simulink model "ControlSystem"  (R2022a)
settings: Solver=FixedStepAuto  StartTime=0.0  StopTime=35  FixedStep=0.01  RelTol=0.01
InitFcn:
  | C=4200;
undefined symbols (not defined in the file): xpoints, ypoints
libraries: simulink_extras x2
settings Model: NumberOfSteps=1100  Creator=tumu  LastModifiedBy=tumu
settings SolverCC: AlgebraicLoopSolver=TrustRegion
settings DebuggingCC: UnconnectedInputMsg=warning  UnconnectedOutputMsg=warning  UnconnectedLineMsg=warning  SFMachineParentedDataDiag=warning  UnderSpecifiedDimensionMsg=warning
settings ModelReferenceCC: ModelReferenceNumInstancesAllowed=Single

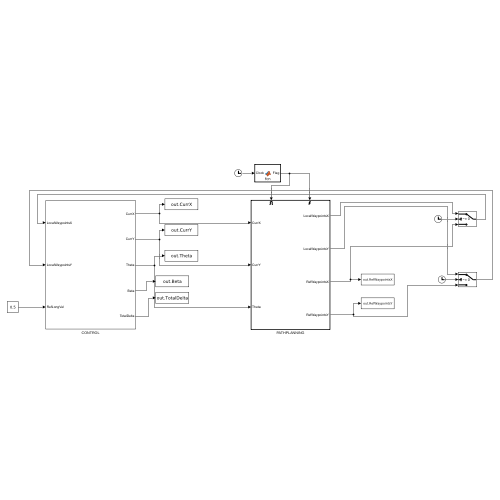
[thumbnail: Simulink's stored preview of the top-level diagram]
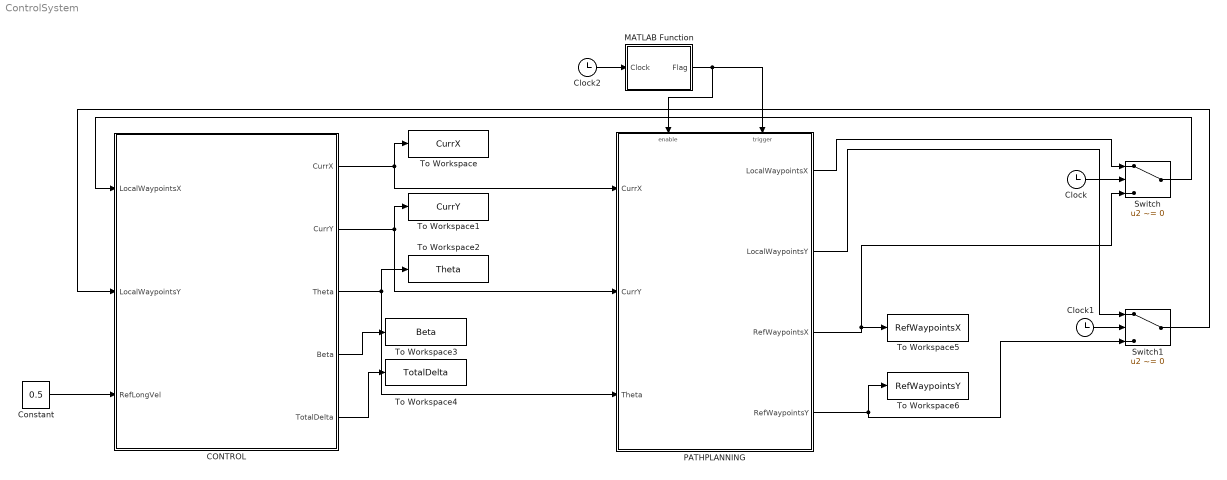
== system ControlSystem ==
  CONTROL : Subsystem
  Clock : Clock
  Clock1 : Clock
  Clock2 : Clock
  Constant : Constant  Value=0.5
  MATLAB Function : MATLAB Function  TreatAsAtomicUnit=on
  PATHPLANNING : Subsystem
  Switch : Switch  Criteria=u2 ~= 0  SaturateOnIntegerOverflow=off  InputSameDT=off
  Switch1 : Switch  Criteria=u2 ~= 0  SaturateOnIntegerOverflow=off  InputSameDT=off
  To Workspace : ToWorkspace  VariableName=CurrX  SaveFormat=Structure With Time  SampleTime=-1
  To Workspace1 : ToWorkspace  VariableName=CurrY  SaveFormat=Structure With Time  SampleTime=-1
  To Workspace2 : ToWorkspace  VariableName=Theta  SaveFormat=Structure With Time  SampleTime=-1
  To Workspace3 : ToWorkspace  VariableName=Beta  SaveFormat=Structure With Time  SampleTime=-1
  To Workspace4 : ToWorkspace  VariableName=TotalDelta  SaveFormat=Structure With Time  SampleTime=-1
  To Workspace5 : ToWorkspace  VariableName=RefWaypointsX  SampleTime=-1
      settings: Save2DSignal=2-D array (concatenate along first dimension)
  To Workspace6 : ToWorkspace  VariableName=RefWaypointsY  SampleTime=-1
      settings: Save2DSignal=2-D array (concatenate along first dimension)
  wires:
  CONTROL/2(CurrY) -> To Workspace1/1, PATHPLANNING/2(CurrY)
  CONTROL/3(Theta) -> To Workspace2/1, PATHPLANNING/3(Theta)
  CONTROL/4(Beta) -> To Workspace3/1
  CONTROL/5(TotalDelta) -> To Workspace4/1
  CONTROL/1(CurrX) -> To Workspace/1, PATHPLANNING/1(CurrX)
  PATHPLANNING/1(LocalWaypointsX) -> Switch/1
  Clock2/1 -> MATLAB Function/1(Clock)
  MATLAB Function/1(Flag) -> PATHPLANNING/Trigger, PATHPLANNING/Enable
  PATHPLANNING/3(RefWaypointsX) -> To Workspace5/1, Switch/3
  PATHPLANNING/4(RefWaypointsY) -> Switch1/3, To Workspace6/1
  Clock/1 -> Switch/2
  Switch/1 -> CONTROL/1(LocalWaypointsX)
  Clock1/1 -> Switch1/2
  Switch1/1 -> CONTROL/2(LocalWaypointsY)
  PATHPLANNING/2(LocalWaypointsY) -> Switch1/1
  Constant/1 -> CONTROL/3(RefLongVel)

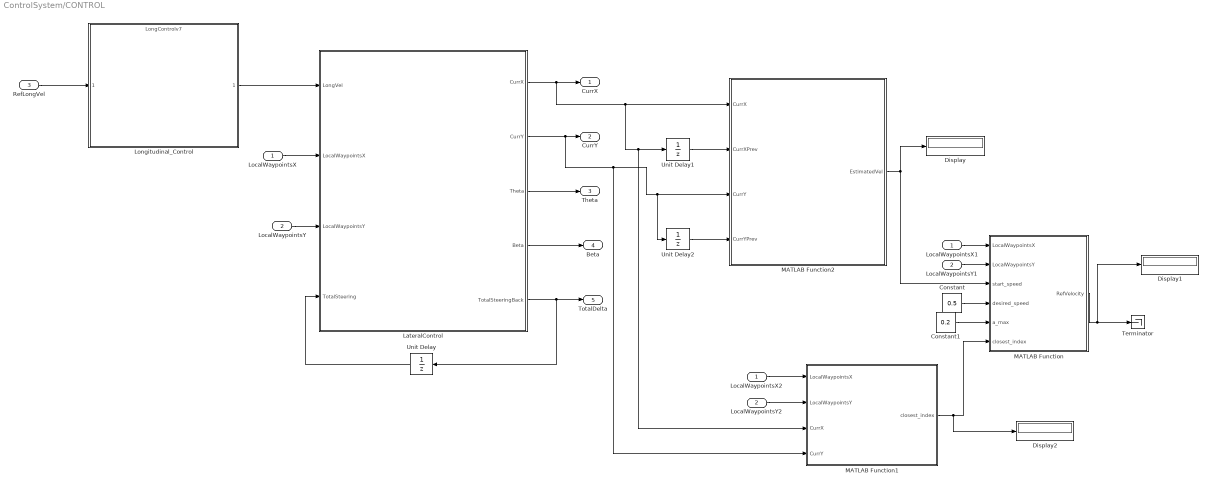
== system ControlSystem/CONTROL ==
  LocalWaypointsX : Inport
  LocalWaypointsY : Inport  Port=2
  RefLongVel : Inport  Port=3
  Constant : Constant  Value=0.5
  Constant1 : Constant  Value=0.2
  Display : Display
  Display1 : Display
  Display2 : Display
  LateralControl : Subsystem
  LocalWaypointsX1 : InportShadow
  LocalWaypointsX2 : InportShadow
  LocalWaypointsY1 : InportShadow  Port=2
  LocalWaypointsY2 : InportShadow  Port=2
  Longitudinal_Control : ModelReference  ModelNameDialog=LongControlv7.slx  SimulationMode=Normal  ModelReferenceVersion=1.48
  MATLAB Function : MATLAB Function  TreatAsAtomicUnit=on
  MATLAB Function1 : MATLAB Function  TreatAsAtomicUnit=on
  MATLAB Function2 : MATLAB Function  TreatAsAtomicUnit=on
  Terminator : Terminator
  Unit Delay : UnitDelay  SampleTime=-1  HasFrameUpgradeWarning=on
  Unit Delay1 : UnitDelay  SampleTime=-1  HasFrameUpgradeWarning=on
  Unit Delay2 : UnitDelay  InitialCondition=1  SampleTime=-1  HasFrameUpgradeWarning=on
  CurrX : Outport
  CurrY : Outport  Port=2
  Theta : Outport  Port=3
  Beta : Outport  Port=4
  TotalDelta : Outport  Port=5
  wires:
  LateralControl/4(Beta) -> Beta/1
  LateralControl/2(CurrY) -> MATLAB Function1/4(CurrY), Unit Delay2/1, MATLAB Function2/3(CurrY), CurrY/1
  LateralControl/1(CurrX) -> MATLAB Function1/3(CurrX), Unit Delay1/1, MATLAB Function2/1(CurrX), CurrX/1
  Unit Delay/1 -> LateralControl/4(TotalSteering)
  LocalWaypointsX/1 -> LateralControl/2(LocalWaypointsX)
  LocalWaypointsY/1 -> LateralControl/3(LocalWaypointsY)
  LateralControl/3(Theta) -> Theta/1
  LateralControl/5(TotalSteeringBack) -> TotalDelta/1, Unit Delay/1
  RefLongVel/1 -> Longitudinal_Control/1
  Longitudinal_Control/1 -> LateralControl/1(LongVel)
  Unit Delay1/1 -> MATLAB Function2/2(CurrXPrev)
  Unit Delay2/1 -> MATLAB Function2/4(CurrYPrev)
  MATLAB Function2/1(EstimatedVel) -> MATLAB Function/3(start_speed), Display/1
  Constant/1 -> MATLAB Function/4(desired_speed)
  Constant1/1 -> MATLAB Function/5(a_max)
  MATLAB Function1/1(closest_index) -> Display2/1, MATLAB Function/6(closest_index)
  LocalWaypointsX1/1 -> MATLAB Function/1(LocalWaypointsX)
  LocalWaypointsX2/1 -> MATLAB Function1/1(LocalWaypointsX)
  LocalWaypointsY1/1 -> MATLAB Function/2(LocalWaypointsY)
  LocalWaypointsY2/1 -> MATLAB Function1/2(LocalWaypointsY)
  MATLAB Function/1(RefVelocity) -> Terminator/1, Display1/1

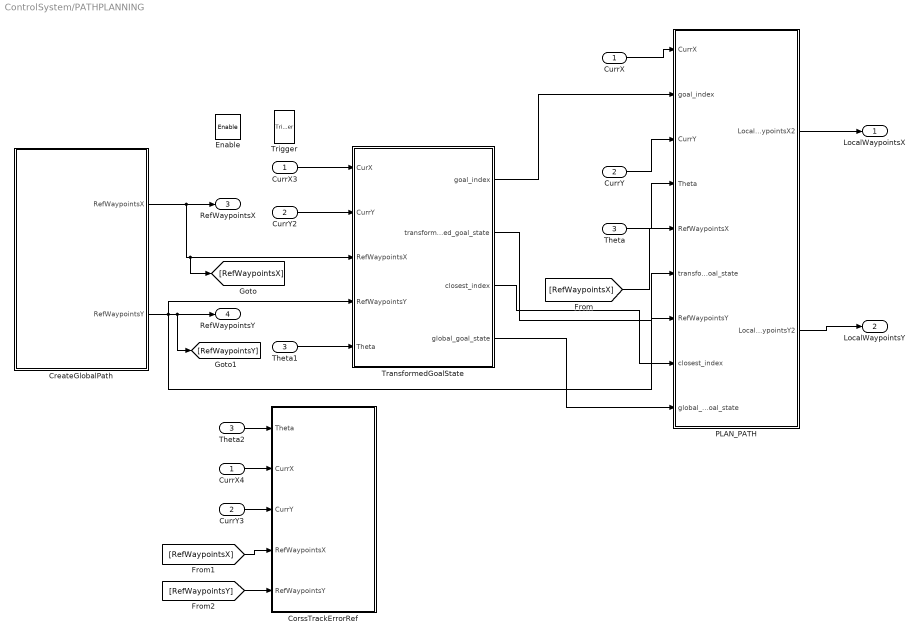
== system ControlSystem/PATHPLANNING ==
  CurrX : Inport
  CurrY : Inport  Port=2
  Theta : Inport  Port=3
  Enable : EnablePort
  Trigger : TriggerPort  VariantControl=Variant  PortDimensions=1
  CorssTrackErrorRef : Subsystem
  CreateGlobalPath : Subsystem
  CurrX3 : InportShadow
  CurrX4 : InportShadow
  CurrY2 : InportShadow  Port=2
  CurrY3 : InportShadow  Port=2
  PLAN_PATH : Subsystem
  Theta1 : InportShadow  Port=3
  Theta2 : InportShadow  Port=3
  TransformedGoalState : Subsystem
  LocalWaypointsX : Outport  PortDimensions=[1 2600]  InitialOutput=[0.01:0.01:26]
  LocalWaypointsY : Outport  Port=2  PortDimensions=[1 2600]  InitialOutput=[ones(1,2600)]
  RefWaypointsX : Outport  Port=3  InitialOutput=[0.01:0.01:26]
  RefWaypointsY : Outport  Port=4  InitialOutput=[ones(1,2600)]
  wires:
  Theta2/1 -> CorssTrackErrorRef/1(Theta)
  CurrX4/1 -> CorssTrackErrorRef/2(CurrX)
  CurrY3/1 -> CorssTrackErrorRef/3(CurrY)
  CurrX3/1 -> TransformedGoalState/1(CurX)
  CurrY2/1 -> TransformedGoalState/2(CurrY)
  Theta1/1 -> TransformedGoalState/5(Theta)
  Theta/1 -> PLAN_PATH/4(Theta)
  TransformedGoalState/2(transformed_goal_state) -> PLAN_PATH/6(transformed_goal_state)
  TransformedGoalState/1(goal_index) -> PLAN_PATH/2(goal_index)
  PLAN_PATH/1(LocalWaypointsX2) -> LocalWaypointsX/1
  PLAN_PATH/2(LocalWaypointsY2) -> LocalWaypointsY/1
  CurrY/1 -> PLAN_PATH/3(CurrY)
  CurrX/1 -> PLAN_PATH/1(CurrX)
  [RefWaypointsX] -> CorssTrackErrorRef/4(RefWaypointsX)
  [RefWaypointsY] -> CorssTrackErrorRef/5(RefWaypointsY)
  CreateGlobalPath/1(RefWaypointsX) -> [RefWaypointsX], TransformedGoalState/3(RefWaypointsX), RefWaypointsX/1
  CreateGlobalPath/2(RefWaypointsY) -> TransformedGoalState/4(RefWaypointsY), PLAN_PATH/7(RefWaypointsY), [RefWaypointsY], RefWaypointsY/1
  [RefWaypointsX] -> PLAN_PATH/5(RefWaypointsX)
  TransformedGoalState/3(closest_index) -> PLAN_PATH/8(closest_index)
  TransformedGoalState/4(global_goal_state) -> PLAN_PATH/9(global_goal_state)

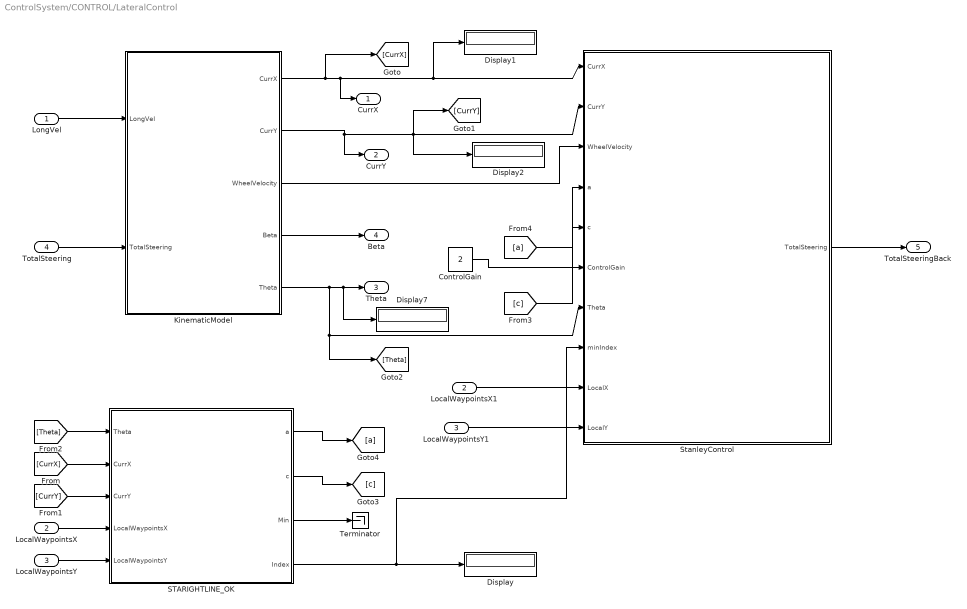
== system ControlSystem/CONTROL/LateralControl ==
  LongVel : Inport
  LocalWaypointsX : Inport  Port=2
  LocalWaypointsY : Inport  Port=3
  TotalSteering : Inport  Port=4
  ControlGain : Constant  Value=2
  Display{,1..2,7} (4 alike) : Display
  KinematicModel : Subsystem
  LocalWaypointsX1 : InportShadow  Port=2
  LocalWaypointsY1 : InportShadow  Port=3
  STARIGHTLINE_OK : MATLAB Function  TreatAsAtomicUnit=on
  StanleyControl : Subsystem
  Terminator : Terminator
  CurrX : Outport
  CurrY : Outport  Port=2
  Theta : Outport  Port=3
  Beta : Outport  Port=4
  TotalSteeringBack : Outport  Port=5
  wires:
  LongVel/1 -> KinematicModel/1(LongVel)
  TotalSteering/1 -> KinematicModel/2(TotalSteering)
  KinematicModel/1(CurrX) -> [CurrX], CurrX/1, Display1/1, StanleyControl/1(CurrX)
  KinematicModel/2(CurrY) -> CurrY/1, Display2/1, [CurrY], StanleyControl/2(CurrY)
  KinematicModel/5(Theta) -> [Theta], StanleyControl/7(Theta), Display7/1, Theta/1
  KinematicModel/4(Beta) -> Beta/1
  KinematicModel/3(WheelVelocity) -> StanleyControl/3(WheelVelocity)
  StanleyControl/1(TotalSteering) -> TotalSteeringBack/1
  ControlGain/1 -> StanleyControl/6(ControlGain)
  LocalWaypointsX/1 -> STARIGHTLINE_OK/4(LocalWaypointsX)
  LocalWaypointsY/1 -> STARIGHTLINE_OK/5(LocalWaypointsY)
  [CurrX] -> STARIGHTLINE_OK/2(CurrX)
  [CurrY] -> STARIGHTLINE_OK/3(CurrY)
  [Theta] -> STARIGHTLINE_OK/1(Theta)
  STARIGHTLINE_OK/2(c) -> [c]
  [c] -> StanleyControl/5(c)
  STARIGHTLINE_OK/1(a) -> [a]
  [a] -> StanleyControl/4(a)
  STARIGHTLINE_OK/3(Min) -> Terminator/1
  STARIGHTLINE_OK/4(Index) -> StanleyControl/8(minIndex), Display/1
  LocalWaypointsX1/1 -> StanleyControl/9(LocalX)
  LocalWaypointsY1/1 -> StanleyControl/10(LocalY)

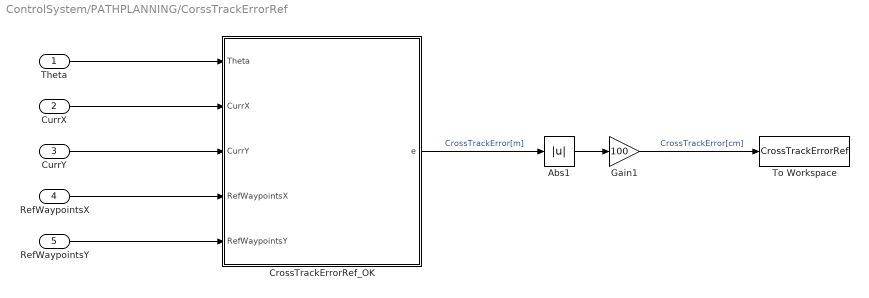
== system ControlSystem/PATHPLANNING/CorssTrackErrorRef ==
  Theta : Inport
  CurrX : Inport  Port=2
  CurrY : Inport  Port=3
  RefWaypointsX : Inport  Port=4
  RefWaypointsY : Inport  Port=5
  Abs1 : Abs  SaturateOnIntegerOverflow=off
  CrossTrackErrorRef_OK : MATLAB Function  TreatAsAtomicUnit=on
  Gain1 : Gain  Gain=100
  To Workspace : ToWorkspace  VariableName=CrossTrackErrorRef  SaveFormat=Structure With Time  SampleTime=-1
  wires:
  CurrX/1 -> CrossTrackErrorRef_OK/2(CurrX)
  Gain1/1 -> To Workspace/1  "CrossTrackError[cm]"
  CrossTrackErrorRef_OK/1(e) -> Abs1/1  "CrossTrackError[m]"
  Abs1/1 -> Gain1/1
  CurrY/1 -> CrossTrackErrorRef_OK/3(CurrY)
  RefWaypointsY/1 -> CrossTrackErrorRef_OK/5(RefWaypointsY)
  Theta/1 -> CrossTrackErrorRef_OK/1(Theta)
  RefWaypointsX/1 -> CrossTrackErrorRef_OK/4(RefWaypointsX)

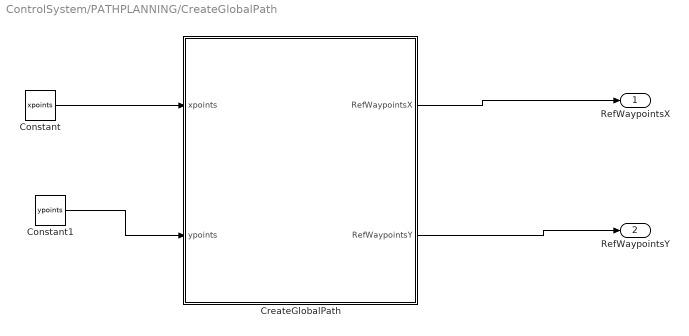
== system ControlSystem/PATHPLANNING/CreateGlobalPath ==
  Constant : Constant  Value=xpoints
  Constant1 : Constant  Value=ypoints
  CreateGlobalPath : MATLAB Function  TreatAsAtomicUnit=on
  RefWaypointsX : Outport  InitialOutput=[0.01:0.01:50]
  RefWaypointsY : Outport  Port=2
  wires:
  CreateGlobalPath/2(RefWaypointsY) -> RefWaypointsY/1
  CreateGlobalPath/1(RefWaypointsX) -> RefWaypointsX/1
  Constant/1 -> CreateGlobalPath/1(xpoints)
  Constant1/1 -> CreateGlobalPath/2(ypoints)

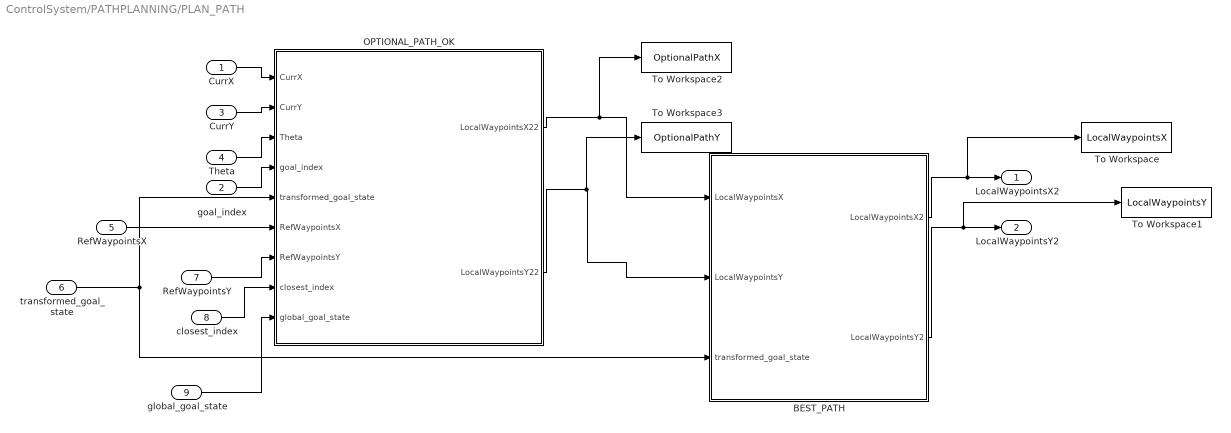
== system ControlSystem/PATHPLANNING/PLAN_PATH ==
  CurrX : Inport
  goal_index : Inport  Port=2
  CurrY : Inport  Port=3
  Theta : Inport  Port=4
  RefWaypointsX : Inport  Port=5
  transformed_goal_state : Inport  Port=6
  RefWaypointsY : Inport  Port=7
  closest_index : Inport  Port=8  PortDimensions=1
  global_goal_state : Inport  Port=9  PortDimensions=[7 3]
  BEST_PATH : MATLAB Function  TreatAsAtomicUnit=on
  OPTIONAL_PATH_OK : MATLAB Function  TreatAsAtomicUnit=on
  To Workspace : ToWorkspace  VariableName=LocalWaypointsX  SampleTime=-1
      settings: Save2DSignal=2-D array (concatenate along first dimension)
  To Workspace1 : ToWorkspace  VariableName=LocalWaypointsY  SampleTime=-1
      settings: Save2DSignal=2-D array (concatenate along first dimension)
  To Workspace2 : ToWorkspace  VariableName=OptionalPathX  SaveFormat=Structure With Time  SampleTime=-1
      settings: Save2DSignal=2-D array (concatenate along first dimension)
  To Workspace3 : ToWorkspace  VariableName=OptionalPathY  SaveFormat=Structure With Time  SampleTime=-1
      settings: Save2DSignal=2-D array (concatenate along first dimension)
  LocalWaypointsX2 : Outport
  LocalWaypointsY2 : Outport  Port=2
  wires:
  CurrX/1 -> OPTIONAL_PATH_OK/1(CurrX)
  CurrY/1 -> OPTIONAL_PATH_OK/2(CurrY)
  RefWaypointsX/1 -> OPTIONAL_PATH_OK/6(RefWaypointsX)
  BEST_PATH/1(LocalWaypointsX2) -> To Workspace/1, LocalWaypointsX2/1
  transformed_goal_state/1 -> BEST_PATH/3(transformed_goal_state), OPTIONAL_PATH_OK/5(transformed_goal_state)
  OPTIONAL_PATH_OK/2(LocalWaypointsY22) -> To Workspace3/1, BEST_PATH/2(LocalWaypointsY)
  goal_index/1 -> OPTIONAL_PATH_OK/4(goal_index)
  BEST_PATH/2(LocalWaypointsY2) -> LocalWaypointsY2/1, To Workspace1/1
  OPTIONAL_PATH_OK/1(LocalWaypointsX22) -> To Workspace2/1, BEST_PATH/1(LocalWaypointsX)
  Theta/1 -> OPTIONAL_PATH_OK/3(Theta)
  RefWaypointsY/1 -> OPTIONAL_PATH_OK/7(RefWaypointsY)
  closest_index/1 -> OPTIONAL_PATH_OK/8(closest_index)
  global_goal_state/1 -> OPTIONAL_PATH_OK/9(global_goal_state)

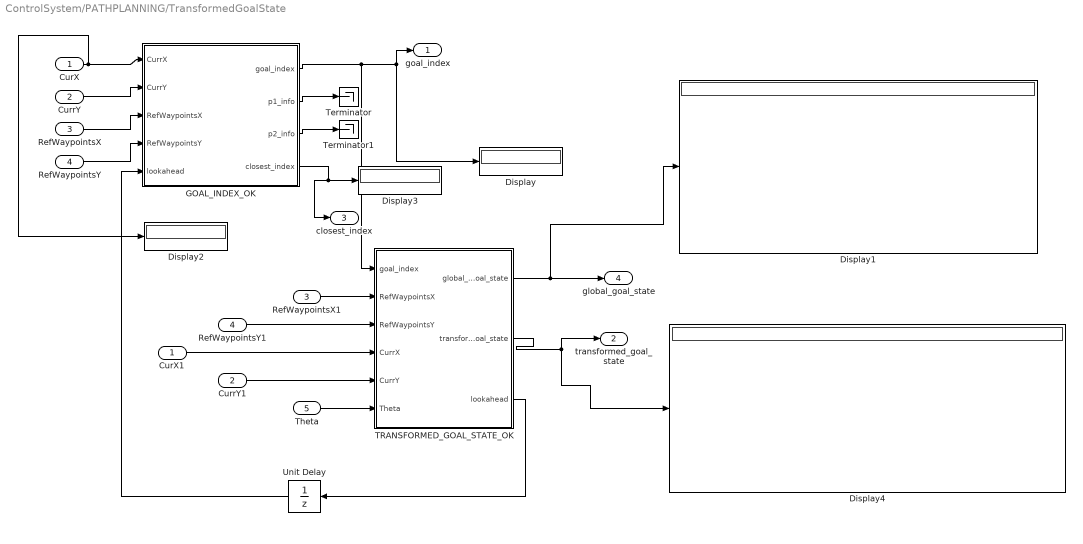
== system ControlSystem/PATHPLANNING/TransformedGoalState ==
  CurX : Inport
  CurrY : Inport  Port=2
  RefWaypointsX : Inport  Port=3
  RefWaypointsY : Inport  Port=4
  Theta : Inport  Port=5
  CurX1 : InportShadow
  CurrY1 : InportShadow  Port=2
  Display{,1..4} (5 alike) : Display
  GOAL_INDEX_OK : MATLAB Function  TreatAsAtomicUnit=on
  RefWaypointsX1 : InportShadow  Port=3
  RefWaypointsY1 : InportShadow  Port=4
  TRANSFORMED_GOAL_STATE_OK : MATLAB Function  TreatAsAtomicUnit=on
  Terminator : Terminator
  Terminator1 : Terminator
  Unit Delay : UnitDelay  InitialCondition=0.5  SampleTime=-1  HasFrameUpgradeWarning=on
  goal_index : Outport
  transformed_goal_state : Outport  Port=2
  closest_index : Outport  Port=3
  global_goal_state : Outport  Port=4
  wires:
  RefWaypointsY1/1 -> TRANSFORMED_GOAL_STATE_OK/3(RefWaypointsY)
  TRANSFORMED_GOAL_STATE_OK/1(global_goal_state) -> global_goal_state/1, Display1/1
  RefWaypointsX/1 -> GOAL_INDEX_OK/3(RefWaypointsX)
  GOAL_INDEX_OK/1(goal_index) -> TRANSFORMED_GOAL_STATE_OK/1(goal_index), Display/1, goal_index/1
  CurrY/1 -> GOAL_INDEX_OK/2(CurrY)
  GOAL_INDEX_OK/3(p2_info) -> Terminator1/1
  RefWaypointsX1/1 -> TRANSFORMED_GOAL_STATE_OK/2(RefWaypointsX)
  GOAL_INDEX_OK/2(p1_info) -> Terminator/1
  RefWaypointsY/1 -> GOAL_INDEX_OK/4(RefWaypointsY)
  Theta/1 -> TRANSFORMED_GOAL_STATE_OK/6(Theta)
  CurrY1/1 -> TRANSFORMED_GOAL_STATE_OK/5(CurrY)
  CurX1/1 -> TRANSFORMED_GOAL_STATE_OK/4(CurrX)
  GOAL_INDEX_OK/4(closest_index) -> Display3/1, closest_index/1
  CurX/1 -> Display2/1, GOAL_INDEX_OK/1(CurrX)
  TRANSFORMED_GOAL_STATE_OK/2(transformed_goal_state) -> Display4/1, transformed_goal_state/1
  TRANSFORMED_GOAL_STATE_OK/3(lookahead) -> Unit Delay/1
  Unit Delay/1 -> GOAL_INDEX_OK/5(lookahead)

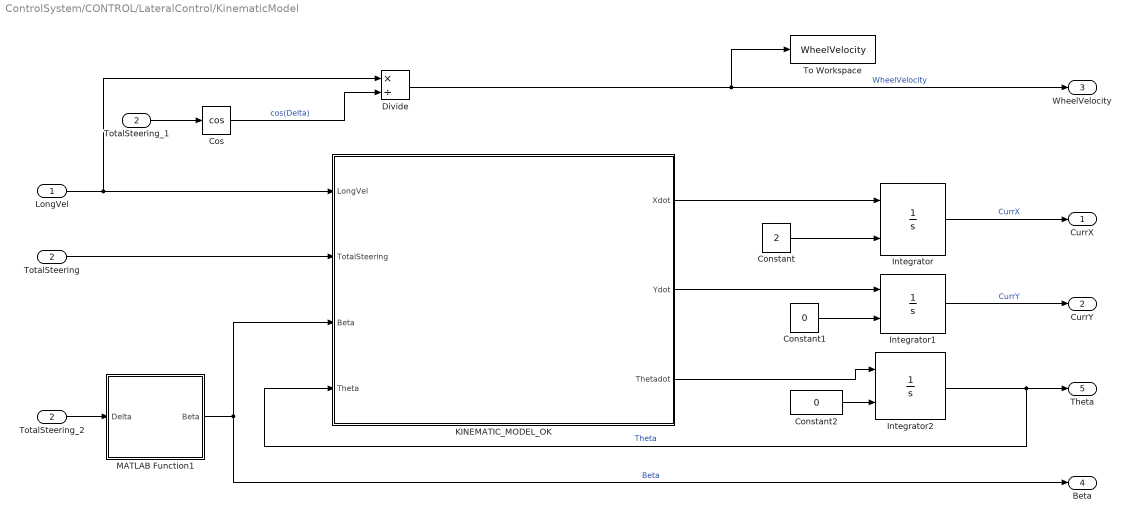
== system ControlSystem/CONTROL/LateralControl/KinematicModel ==
  LongVel : Inport
  TotalSteering : Inport  Port=2
  Constant : Constant  Value=2
  Constant1 : Constant  Value=0
  Constant2 : Constant  Value=0
  Cos : Trigonometry  Operator=cos
  Divide : Product  Inputs=*/
  Integrator : Integrator  InitialConditionSource=external
  Integrator1 : Integrator  InitialConditionSource=external
  Integrator2 : Integrator  InitialConditionSource=external
  KINEMATIC_MODEL_OK : MATLAB Function  TreatAsAtomicUnit=on
  MATLAB Function1 : MATLAB Function  TreatAsAtomicUnit=on
  To Workspace : ToWorkspace  VariableName=WheelVelocity  SaveFormat=Structure With Time  SampleTime=-1
  TotalSteering_1 : InportShadow  Port=2
  TotalSteering_2 : InportShadow  Port=2
  CurrX : Outport
  CurrY : Outport  Port=2
  WheelVelocity : Outport  Port=3
  Beta : Outport  Port=4
  Theta : Outport  Port=5
  wires:
  KINEMATIC_MODEL_OK/3(Thetadot) -> Integrator2/1
  TotalSteering_2/1 -> MATLAB Function1/1(Delta)
  KINEMATIC_MODEL_OK/2(Ydot) -> Integrator1/1
  TotalSteering/1 -> KINEMATIC_MODEL_OK/2(TotalSteering)
  Constant2/1 -> Integrator2/2
  Divide/1 -> To Workspace/1, WheelVelocity/1  "WheelVelocity"
  MATLAB Function1/1(Beta) -> Beta/1, KINEMATIC_MODEL_OK/3(Beta)  "Beta"
  LongVel/1 -> Divide/1, KINEMATIC_MODEL_OK/1(LongVel)
  Integrator2/1 -> Theta/1, KINEMATIC_MODEL_OK/4(Theta)  "Theta"
  Integrator/1 -> CurrX/1  "CurrX"
  KINEMATIC_MODEL_OK/1(Xdot) -> Integrator/1
  Constant/1 -> Integrator/2
  TotalSteering_1/1 -> Cos/1
  Integrator1/1 -> CurrY/1  "CurrY"
  Cos/1 -> Divide/2  "cos(Delta)"
  Constant1/1 -> Integrator1/2

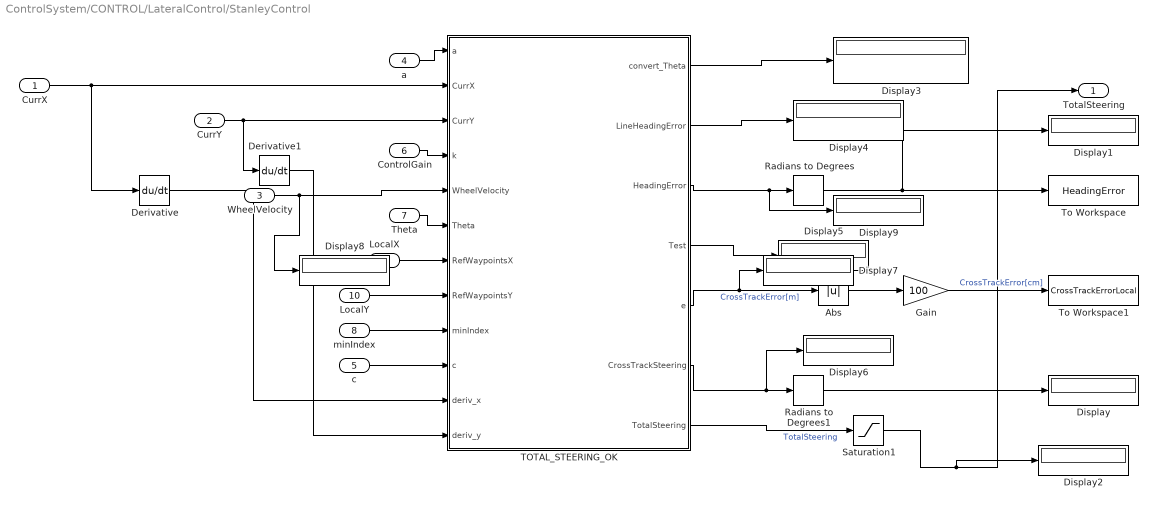
== system ControlSystem/CONTROL/LateralControl/StanleyControl ==
  CurrX : Inport
  CurrY : Inport  Port=2
  WheelVelocity : Inport  Port=3
  a : Inport  Port=4
  c : Inport  Port=5
  ControlGain : Inport  Port=6
  Theta : Inport  Port=7
  minIndex : Inport  Port=8
  LocalX : Inport  Port=9
  LocalY : Inport  Port=10
  Abs : Abs  SaturateOnIntegerOverflow=off
  Derivative : Derivative
  Derivative1 : Derivative
  Display{,1..9} (10 alike) : Display
  Gain : Gain  Gain=100
  Radians to Degrees : simulink_extras/Transformations/Radians to Degrees
  Radians to Degrees1 : simulink_extras/Transformations/Radians to Degrees
  Saturation1 : Saturate  UpperLimit=1  LowerLimit=-1
  TOTAL_STEERING_OK : MATLAB Function  TreatAsAtomicUnit=on
  To Workspace : ToWorkspace  VariableName=HeadingError  SaveFormat=Structure With Time  SampleTime=-1
  To Workspace1 : ToWorkspace  VariableName=CrossTrackErrorLocal  SaveFormat=Structure With Time  SampleTime=-1
  TotalSteering : Outport
  wires:
  CurrY/1 -> Derivative1/1, TOTAL_STEERING_OK/3(CurrY)
  CurrX/1 -> Derivative/1, TOTAL_STEERING_OK/2(CurrX)
  a/1 -> TOTAL_STEERING_OK/1(a)
  c/1 -> TOTAL_STEERING_OK/10(c)
  WheelVelocity/1 -> Display8/1, TOTAL_STEERING_OK/5(WheelVelocity)
  ControlGain/1 -> TOTAL_STEERING_OK/4(k)
  TOTAL_STEERING_OK/7(TotalSteering) -> Saturation1/1  "TotalSteering"
  Saturation1/1 -> TotalSteering/1, Display2/1
  Theta/1 -> TOTAL_STEERING_OK/6(Theta)
  TOTAL_STEERING_OK/3(HeadingError) -> Display9/1, Radians to Degrees/1
  TOTAL_STEERING_OK/5(e) -> Display7/1, Abs/1  "CrossTrackError[m]"
  Abs/1 -> Gain/1
  Gain/1 -> To Workspace1/1  "CrossTrackError[cm]"
  Radians to Degrees/1 -> Display1/1, To Workspace/1
  TOTAL_STEERING_OK/6(CrossTrackSteering) -> Display6/1, Radians to Degrees1/1
  Radians to Degrees1/1 -> Display/1
  minIndex/1 -> TOTAL_STEERING_OK/9(minIndex)
  Derivative/1 -> TOTAL_STEERING_OK/11(deriv_x)
  Derivative1/1 -> TOTAL_STEERING_OK/12(deriv_y)
  LocalY/1 -> TOTAL_STEERING_OK/8(RefWaypointsY)
  LocalX/1 -> TOTAL_STEERING_OK/7(RefWaypointsX)
  TOTAL_STEERING_OK/1(convert_Theta) -> Display3/1
  TOTAL_STEERING_OK/2(LineHeadingError) -> Display4/1
  TOTAL_STEERING_OK/4(Test) -> Display5/1

== matlab function ControlSystem/CONTROL/MATLAB Function1 ==
  data: LocalWaypointsX input; closest_index output; LocalWaypointsY input; CurrX input; CurrY input
function closest_index = fcn(LocalWaypointsX,LocalWaypointsY,CurrX,CurrY)

Distance = zeros(1,length(LocalWaypointsX));
for i=1:1:length(LocalWaypointsX)
    Distance(1,i)= sqrt((CurrX-LocalWaypointsX(i))^2+(CurrY-LocalWaypointsY(i))^2);
       
end

[~,closest_index]=min(Distance); % Min distance from Current position of front wheel to the path.

== matlab function ControlSystem/PATHPLANNING/PLAN_PATH/BEST_PATH ==
  data: LocalWaypointsX input; LocalWaypointsX2 output; LocalWaypointsY input; transformed_goal_state input; LocalWaypointsY2 output
function [LocalWaypointsX2,LocalWaypointsY2] = fcn(LocalWaypointsX,LocalWaypointsY,transformed_goal_state)
CenterX = 6;
CenterY = 0.25;
Radius = 0.1;
num_paths = 7;
NumberofWaypoints=2600;
DistanceCenter = zeros(1,NumberofWaypoints,num_paths);
DistanceGoal = zeros(1,NumberofWaypoints,num_paths);
path_validity = ones(num_paths,1);
Objective = zeros(1,num_paths);
LocalWaypointsX2 = zeros(1,NumberofWaypoints);
LocalWaypointsY2 = zeros(1,NumberofWaypoints);
best_index = round(num_paths/2);
best_index_score = 0.1;
DistanceCheck = zeros(1,num_paths);
    for j=1:1:num_paths
        for i=1:1:NumberofWaypoints
            DistanceCenter(1,i,j) = sqrt((LocalWaypointsX(1,i,j)-CenterX)^2+(LocalWaypointsY(1,i,j)-CenterY)^2); 
            DistanceGoal(1,i,j) = sqrt((LocalWaypointsX(1,i,j)-transformed_goal_state(round(num_paths/2),1))^2+(LocalWaypointsY(1,i,j)-transformed_goal_state(round(num_paths/2),2))^2); 
        end
    end
DistanceGoal(:,:,1)=DistanceGoal(:,:,1)*1.8;
DistanceGoal(:,:,2)=DistanceGoal(:,:,2)*1.7;
DistanceGoal(:,:,3)=DistanceGoal(:,:,3)*1.5;
DistanceGoal(:,:,4)=DistanceGoal(:,:,4)*1;
DistanceGoal(:,:,5)=DistanceGoal(:,:,5)*1.2;
DistanceGoal(:,:,6)=DistanceGoal(:,:,6)*1.3;
DistanceGoal(:,:,7)=DistanceGoal(:,:,7)*1.4;

    for j=1:1:num_paths
        DistanceCheck(1,j)= min(DistanceCenter(:,:,j));
        Objective(1,j) = sum(DistanceGoal(:,:,j));
        if DistanceCheck(1,j) < Radius
            path_validity(j) = 0;
        end
    end
Observe = Objective;
    for j=1:1:num_paths
        [Min,I] = min(Objective);
        Objective(I) = nan;
        if path_validity(I)==1
            best_index = I;
            break; 
        end
    end

LocalWaypointsX2 = LocalWaypointsX(1,:,best_index);
LocalWaypointsY2 = LocalWaypointsY(1,:,best_index);

== matlab function ControlSystem/PATHPLANNING/PLAN_PATH/OPTIONAL_PATH_OK ==
  data: CurrX input; LocalWaypointsX22 output size=[1 2600 7]; CurrY input; Theta input; goal_index input; transformed_goal_state input; RefWaypointsX input; LocalWaypointsY22 output size=[1 2600 7]; RefWaypointsY input; closest_index input; global_goal_state input
function [LocalWaypointsX22, LocalWaypointsY22] = fcn(CurrX,CurrY,Theta,goal_index,transformed_goal_state,RefWaypointsX,RefWaypointsY,closest_index, global_goal_state)
% function [LocalWaypointsX, LocalWaypointsY] =
% fcn(CurrX,CurrY,Theta,transformed_goal_state,goal_index,RefWaypointsX)
% creates optional path using transformed_goal_state
% Transformed_goal_state: [x_points y_points heading]   num_pathsx3

%% args:
        % CurrX [m]: Current x posiiton of the vehicle
        % CurrY [m]: Current y poisiton of the vehicle
        % Theta [rad]: Yaw angle
        % goal_index : Goal index on the REF PATH, is needed to create a local path
        % Transformed_goal_state: [x_points y_points heading]   num_pathsx3
        % RefWaypointsX: Ref Path 
%% outputs:
        % LocalWaypointsX: Optional x-path
        % LocalWaypointsY: Optional y-path
NumberofWaypoints=2600;
X = transformed_goal_state(:,1); % goal_state_X point 
Y = transformed_goal_state(:,2); % goal_state_Y point
theta = transformed_goal_state(:,3); % goal_state_Theta
global_goal_state_theta = atan(tan(global_goal_state(:,3)));
theta = tan(theta);
coefficient = zeros(size(transformed_goal_state,1),4);
    if Theta <0.0001 && Theta >-0.0001
        Theta = 0;
    end

%% CALCULTES THE REQUIRED COEFFICIENT
    for i=1:1:size(transformed_goal_state,1)

    A = [X(i)*X(i)*X(i) X(i)*X(i) X(i) 1;0 0 0 1;3*X(i)*X(i) 2*X(i) 1 0;0 0 1 0];
    B = [Y(i);0;theta(i);0];
    coefficient(i,:) = (A\B)';
    end
%% CALCULTES WAYPOINTS OF ALL PATHS

coefficient = coefficient';
coefficient = reshape(coefficient,[1,4,size(transformed_goal_state,1)]); % 1x4x5
LocalWaypointsX = zeros(1,NumberofWaypoints,size(transformed_goal_state,1));
LocalWaypointsX22 = zeros(1,NumberofWaypoints,size(transformed_goal_state,1));
LocalWaypointsY = zeros(1,NumberofWaypoints,size(transformed_goal_state,1));
LocalWaypointsY22 = zeros(1,NumberofWaypoints,size(transformed_goal_state,1));
%TestVehiclePathY = zeros(1,NumberofWaypoints);
%TestVehiclePathX = zeros(1,NumberofWaypoints);
theta = atan(theta);
    for i=1:1:size(transformed_goal_state,1)
        if theta(i) == pi/2
            LocalWaypointsX(:,:,i) = linspace(0,X(i),NumberofWaypoints); % 1x100x5
        else
            LocalWaypointsX(:,:,i) = linspace(0,X(i),NumberofWaypoints); % 1x100x5
        end
        
    end
%TestVehiclePathX(1,:) = LocalWaypointsX(:,:,4);
X_vectorized = [LocalWaypointsX.^3;LocalWaypointsX.^2;LocalWaypointsX;ones(1,NumberofWaypoints,size(transformed_goal_state,1))]; % 4x100x5
    for i=1:1:size(transformed_goal_state,1)
        if theta(i) == pi/2
            LocalWaypointsY(:,:,i) = linspace(RefWaypointsY(closest_index),RefWaypointsY(goal_index),NumberofWaypoints);
        else
            LocalWaypointsY(:,:,i) = coefficient(:,:,i)*X_vectorized(:,:,i);
        end
%TestVehiclePathY(1,:) = LocalWaypointsY(:,:,4);
    end
    for i=1:1:size(transformed_goal_state,1)
        for j=1:1:NumberofWaypoints
            LocalWaypointsX22(:,j,i) = CurrX + (LocalWaypointsX(:,j,i))*(cos(Theta))-(LocalWaypointsY(:,j,i))*(sin(Theta));
            LocalWaypointsY22(:,j,i) = CurrY + (LocalWaypointsX(:,j,i))*(sin(Theta))+(LocalWaypointsY(:,j,i))*(cos(Theta));
        end
    end
for i=1:1:size(transformed_goal_state,1)
    if abs((global_goal_state_theta(i)-pi/2)) <= 0.0001
       LocalWaypointsX22(:,:,i) = (ones(1,NumberofWaypoints))*(RefWaypointsX(goal_index));
        LocalWaypointsY22(:,:,i) = linspace(RefWaypointsY(closest_index),RefWaypointsY(goal_index),NumberofWaypoints);
    end
end

== matlab function ControlSystem/PATHPLANNING/CorssTrackErrorRef/CrossTrackErrorRef_OK ==
  data: Theta input; e output; CurrX input; CurrY input; RefWaypointsX input; RefWaypointsY input
function e = fcn(Theta,CurrX,CurrY,RefWaypointsX,RefWaypointsY)
% function e = fcn(Theta,CurrX,CurrY,RefWaypointsX,RefWaypointsY)
% calculates the coefficient of straight line and distance to that straigth
% line from front wheel.

Distance = zeros(1,length(RefWaypointsX));

Lf = 0.053; % Distance between c.o.g. and the front wheel
CurrWheelX = CurrX+(Lf)*cos(Theta); % CurrentX position of front wheel w.r.t. Global Frame
CurrWheelY = CurrY+(Lf)*sin(Theta); % CurrentY position of front wheel w.r.t. Global Frame

    for i=1:1:length(RefWaypointsX)
        Distance(1,i)= sqrt((CurrWheelX-RefWaypointsX(i))^2+(CurrWheelY-RefWaypointsY(i))^2);   
    end

[~,Index]=min(Distance); % Min distance from Current position of front wheel to the path.

    if Index==1
        Index=2;
    end

Slope = ((RefWaypointsY(Index))-(RefWaypointsY(Index-1)))/((RefWaypointsX(Index))-(RefWaypointsX(Index-1))); % SLope of the line

a=-Slope;

n=RefWaypointsY(Index)-Slope*RefWaypointsX(Index);
c=-n;

e = abs((a*CurrX+CurrY+c)/(sqrt(a*a+1))); % CrossTrackError [m]

Test = a*CurrX+CurrY+c; % Checks the position of the CurrPoint w.r.t line

    if Test > 0
        e = -e;
    end

== matlab function ControlSystem/PATHPLANNING/TransformedGoalState/GOAL_INDEX_OK ==
  data: CurrX input; goal_index output; CurrY input; RefWaypointsX input; RefWaypointsY input; p1_info output; p2_info output; closest_index output; lookahead input
function [goal_index,p1_info,p2_info,closest_index] = fcn(CurrX,CurrY,RefWaypointsX,RefWaypointsY,lookahead)
% function y = fcn(CurrX,CurrY,RefWaypointsX,RefWaypointsY) calculates the
% goal_index on the path using Lookahead distance.

%% args:
        % CurrX [m]: Current x posiiton of the vehicle
        % CurrY [m]: Current y poisiton of the vehicle
        % RefWaypointsX: Ref Path 
        % RefWaypointsY: Ref Path
%% outputs:
        % goal_index : Goal index on the REF PATH, is needed to create a local path
        % closest_index : Corresponding index on the REF PATH using current
        % posiiton of the vehicle 
%% PRELOCATION
Distance = zeros(1,length(RefWaypointsX));
%lookahead = 0.5; % Lookahead distance [m]
p1_info = 0;
p2_info = 0;
flag = 1;
flag2 = 1;
%% CALCULATES closest length and index
    for i=1:1:length(RefWaypointsX)
        Distance(1,i)= sqrt((CurrX-RefWaypointsX(i))^2+(CurrY-RefWaypointsY(i))^2);
    end

[closest_len,closest_index]=min(Distance); % Min distance from Current position of front wheel to the path.

    if closest_index==1
        closest_index=2;
    end


%% FINDS GOAL_INDEX USING LOOKAHEAD DISTANCE
arc_length = closest_len;
goal_index= closest_index;

    if arc_length > closest_len
        return
    end

    if goal_index==length(RefWaypointsX)
        return
    end
    
    while goal_index < length(RefWaypointsX)-1
        arc_length = arc_length +sqrt((RefWaypointsX(goal_index)-RefWaypointsX(goal_index+1))^2+(RefWaypointsY(goal_index)-RefWaypointsY(goal_index+1))^2);
        while flag
            if arc_length > (lookahead)/3
                p1_info = goal_index;
                flag=0;
            else
                break
            end
        end

        while flag2
            if arc_length > (2*lookahead)/(3)
                p2_info = goal_index;
                flag2 = 0;
            else
                break
            end
        end

        if arc_length > lookahead
            break
        end
        goal_index=goal_index+1;

    end
    
    
end

== matlab function ControlSystem/PATHPLANNING/TransformedGoalState/TRANSFORMED_GOAL_STATE_OK ==
  data: goal_index input; global_goal_state output; RefWaypointsX input; RefWaypointsY input; CurrX input; CurrY input; Theta input; transformed_goal_state output; lookahead output size=1
function [global_goal_state,transformed_goal_state,lookahead] = fcn(goal_index,RefWaypointsX,RefWaypointsY,CurrX,CurrY,Theta)
% function transformed_state_set =
% fcn(goal_index,RefWaypointsX,RefWaypointsY,CurrX,CurrY,Theta) first
% calculates the goal_state_set w.r.t vehicle frame and then transforms
% into Global frame
%% args:
        % goal_index : Goal index on the REF PATH, is needed to create a local path
        % RefWaypointsX: Ref Path 
        % RefWaypointsY: Ref Path
        % CurrX [m]: Current x posiiton of the vehicle
        % CurrY [m]: Current y poisiton of the vehicle
        % Theta [rad]: Yaw angle
%% outputs:        
        % Transformed_goal_state: [x_points y_points heading]   num_pathsx3

num_paths = 7; % Number of paths that will be generated.
transformed_goal_state = zeros(num_paths,3);
path_offset = 0.15;
%% CALCULATES HEADING ANGLE OF THE GOAL POINT
    if goal_index == length(RefWaypointsX)
        goal_index = goal_index - 1;
        delta_x = (RefWaypointsX(goal_index+1))-(RefWaypointsX(goal_index));
        delta_y = (RefWaypointsY(goal_index+1))-(RefWaypointsY(goal_index));
    else
        delta_x = (RefWaypointsX(goal_index+1))-(RefWaypointsX(goal_index));
        delta_y = (RefWaypointsY(goal_index+1))-(RefWaypointsY(goal_index));   
    end

heading = atan(delta_y/delta_x);

%% TRANSLATION AND ROTATION TO HAVE GOAL_STATE_SET W.R.T VEHICLE FRAME

goal_state_localX = RefWaypointsX(goal_index)- CurrX;
goal_state_localY = RefWaypointsY(goal_index)- CurrY;

theta = -Theta;
goal_x = (cos(theta))*(goal_state_localX)-(sin(theta))*(goal_state_localY);
goal_y = (cos(theta))*(goal_state_localY)+(sin(theta))*(goal_state_localX);

goal_t = heading-Theta;

    if goal_t > pi
        goal_t= goal_t-2*pi;
    end

    if goal_t < -pi
        goal_t = goal_t +2*pi;
    end


    for i=1:1:num_paths
        offset = (i-round(num_paths/2))*(path_offset);
        %if offset <0
         %   offset=0;
        %end
        x_offset = (offset)*(cos(goal_t+pi/2));
        y_offset = (offset)*(sin(goal_t+pi/2));
        transformed_goal_state(i,:) = [goal_x+x_offset, goal_y+y_offset, goal_t];
    end
%% TRANSFORMS INTO GLOBAL FRAME
x1 = transformed_goal_state(:,1);
y1 = transformed_goal_state(:,2);
goal_state_set_heading = transformed_goal_state(:,3);

x2 = cos(Theta)*x1-sin(Theta)*y1;
y2 = cos(Theta)*y1+sin(Theta)*x1;

x2 = CurrX+x2;
y2 = CurrY+y2;

heading = goal_state_set_heading+Theta;
convert_heading =atan(tan(heading));
if abs(convert_heading-pi/2) <= 0.00001 
    lookahead = 1;
else
    lookahead=0.5;
end

global_goal_state = [x2 y2 heading];

end

== matlab function ControlSystem/MATLAB Function ==
  data: Clock input; Flag output
function Flag  = fcn(Clock)
Flag = 0;

for i=1:1:1000
   % a = (0.2)*(i-1);
    if mod(Clock,0.25) == 0
        Flag = 1;
        break;
    end
    
end

%for i=1:1:1000
 %   a = (0.3)*(i-1);
  %  if Clock == a
   %     Flag = 1;
    %    break;
    %end
    
%end

%for i=1:1:1000
 %   a = (1.7)*(i-1);
  %  if Clock == a
   %     Flag = 1;
    %    break;
    %end
    
%end


%for i=1:1:1000
 %   a = (2.9)*(i-1);
  %  if Clock == a
   %     Flag = 1;
    %    break;
    %end
    
%end


%for i=1:1:1000
 %   a = (4.1)*(i-1);
  %  if Clock == a
   %     Flag = 1;
    %    break;
    %end
    
%end

%for i=1:1:1000
 %   a = (5.3)*(i-1);
  %  if Clock == a
   %     Flag = 1;
    %    break;
    %end
    
%end

== matlab function ControlSystem/PATHPLANNING/CreateGlobalPath/CreateGlobalPath ==
  data: xpoints input; RefWaypointsX output; RefWaypointsY output; ypoints input
function [RefWaypointsX, RefWaypointsY] = fcn(xpoints, ypoints)


% function [RefWaypointsX,RefWaypointsY] = fcn(xc,yc,thetac,xf,yf,thetaf)
% plots the trafectory from limited number of waypoints.

%% args:
        % (xc): is the x coordinates of the waypoints except the last one [m]
        % [x0 x1 .... xn]
        % (yc):is they coordinates of the waypoints except the last one [m]
        % [y0 y1 ...yn] 
        % (thetac):is the yaw angle of the waypoints except the last [rad]
        % [theta0 theta1 ... thetan]
        % (xf): is the x coordinates of the waypoints except the first one [m]
        % [x0 x1 .... xn]
        % (yf):is they coordinates of the waypoints except the first one [m]
        % [y0 y1 ...yn] 
        % (thetaf):is the yaw angle of the waypoints except the first [rad]
        % [theta0 theta1 ... thetan]
        
%% outputs:
            % RefWaypointsX : x points of the path
            % [x0 x1 ... xn]
            % RefWaypointsY : y points of the path
            % [y0 y1 ... yn]
%% PRELOCATION AND INITIALATION       
slopes = zeros(1,length(xpoints));
coeffs = zeros(1,length(xpoints));
NumberOfSamp= 100;
x = zeros(1,NumberOfSamp);
y = zeros(1,NumberOfSamp);
WaypointsX = zeros(1,(NumberOfSamp)*(length(xpoints)-1));
WaypointsY = zeros(1,(NumberOfSamp)*(length(xpoints)-1));
for i=1:1:length(xpoints)
    if i < length(xpoints)
        slopes(i) = (ypoints(i+1)-ypoints(i))/(xpoints(i+1)-xpoints(i));
    else
        slopes(i) = (ypoints(i)-ypoints(1))/(xpoints(i)-xpoints(1));
    end
     
    if isinf(slopes(i))
        if i < length(xpoints)
            x(1:end) = xpoints(i);
            y = linspace(ypoints(i),ypoints(i+1),NumberOfSamp);
        else
            x(1:end) = xpoints(i);
            y = linspace(ypoints(i),ypoints(1),NumberOfSamp);
        end
        
    else
        if i < length(xpoints)
            coeffs(i) = (ypoints(i+1))-(slopes(i))*(xpoints(i+1));
            x = linspace(xpoints(i),xpoints(i+1),NumberOfSamp);
            y = (slopes(i)).*(x)+coeffs(i);
        else
            coeffs(i) = (ypoints(i))-(slopes(i))*(xpoints(i));
            x = linspace(xpoints(i),xpoints(1),NumberOfSamp);
            y = (slopes(i)).*(x)+coeffs(i);
        end
        
    end
    if i<length(xpoints)
    WaypointsX((NumberOfSamp)*(i-1)+1:(NumberOfSamp)*(i))=x;
     WaypointsY((NumberOfSamp)*(i-1)+1:(NumberOfSamp)*(i))=y;
    end
end

RefWaypointsX = WaypointsX ;
RefWaypointsY = WaypointsY ;

== matlab function ControlSystem/CONTROL/LateralControl/KinematicModel/MATLAB Function1 ==
  data: Delta input; Beta output
function Beta = fcn(Delta)
L = 2;  % Length of the car [m]
Lr = 1.2;  % Distance between the rear axle and cog [m] 

%Beta = atan(((Lr)*(tan(Delta)))/(L)); [rad]
Beta =0;   % No slip condition      [rad]

== matlab function ControlSystem/CONTROL/LateralControl/KinematicModel/KINEMATIC_MODEL_OK ==
  data: LongVel input; Xdot output; TotalSteering input; Beta input; Ydot output; Thetadot output; Theta input
function [Xdot,Ydot,Thetadot] = fcn(LongVel,TotalSteering,Beta,Theta)
% function [Xdot,Ydot,Thetadot] = fcn(LongVel,TotalSteering,Beta,Theta)
% calculates the new position of the ego vehicle

%% args:
        % LongVel [m/s] Longitudinal velocity of the vehicle
        % TotalSteering [rad] Steering angle
        % Beta [rad] Slip angle
        % Theta [rad] Angle between global coor frame and front wheel coor
        % frame
%% outputs:
        % Xdot [m/s] Velocity in global x-axis
        % Ydot [m/s] Velocity in global y-axis
        % Thetadot [rad/s] Angular velocity
        
%L = 2; % Length of the car [m]
L = 0.106; % Length of the ROSBOT [m]

Xdot = (LongVel)*(cos(Theta+Beta)); 
Ydot = (LongVel)*(sin(Theta+Beta)); 
Thetadot = ((LongVel)*(cos(Beta))*(tan(TotalSteering)))/(L);

== matlab function ControlSystem/CONTROL/LateralControl/STARIGHTLINE_OK ==
  data: Theta input; CurrX input; CurrY input; LocalWaypointsX input; a output; LocalWaypointsY input; c output; Min output; Index output
function [a,c,Min,Index] = fcn(Theta, CurrX, CurrY, LocalWaypointsX,LocalWaypointsY)
% function [a,c,Min] = fcn(Theta, CurrX, CurrY,
% LocalWaypointsX,LocalWaypointsY) determines the coefficient of closest straight
% line to the front wheel

%% args:
        % Theta [rad]: Yaw angle w.r.t. GLOBAL FRAME
        % CurrX [m]: Current x position of the vehicle
        % CurrY [m]: Current y position of the vehicle
        % LocalWaypointsX : The x-path created by path planning [1 NumberofWaypoints]
        % LocalWaypointsY : The y-path created by path planning [1 NumberofWaypoints]
        
%% outputs:
        % a,c coefficient of the straight line which is closest to the
        % front wheel
        % Index: Closest index
        % Min : The distance beetween the path and the front wheel
        
Distance = zeros(1,length(LocalWaypointsX));
Lf = 0.053; % Distance between c.o.g. and the front wheel
CurrWheelX = CurrX+(Lf)*cos(Theta); % CurrentX position of front wheel w.r.t. Global Frame
CurrWheelY = CurrY+(Lf)*sin(Theta); % CurrentY position of front wheel w.r.t. Global Frame

for i=1:1:length(LocalWaypointsX)
    Distance(1,i)= sqrt((CurrWheelX-LocalWaypointsX(i))^2+(CurrWheelY-LocalWaypointsY(i))^2);
       
end

[Min,Index]=min(Distance); % Min distance from Current position of front wheel to the path.

if Index==1
    Index=2;
end
if Index == length(LocalWaypointsX)
    Index = Index-1;
end
Slope = ((LocalWaypointsY(Index+1))-(LocalWaypointsY(Index)))/((LocalWaypointsX(Index+1))-(LocalWaypointsX(Index))); % SLope of the line

a=-Slope;

n=LocalWaypointsY(Index+1)-Slope*LocalWaypointsX(Index+1);
c=-n;

== matlab function ControlSystem/CONTROL/LateralControl/StanleyControl/TOTAL_STEERING_OK ==
  data: convert_Theta output; LineHeadingError output; HeadingError output; Test output; e output; CrossTrackSteering output; a input; CurrX input; CurrY input; k input; WheelVelocity input; Theta input; RefWaypointsX input; RefWaypointsY input; minIndex input; c input; TotalSteering output; deriv_x input; deriv_y input
function [convert_Theta,LineHeadingError,HeadingError,Test,e,CrossTrackSteering,TotalSteering]   = fcn(a,CurrX,CurrY,k,WheelVelocity,Theta,RefWaypointsX,RefWaypointsY,minIndex,c,deriv_x,deriv_y)
% a,c coeff of the line
% CurrX [m] Current x position of the vehicle
% CurrY [m] Current y position of the vehicle
% k Control gain
% WheelVel [m/s] Velocity of the wheel in the wheel coor framee
% Theta [rad] Orientation w.r.t Global coor frame

if WheelVelocity==0
    WheelVelocity=0.01;
end
convert_Theta=atan(tan(Theta));

delta_y=RefWaypointsY(minIndex+1)-RefWaypointsY(minIndex);
delta_x=RefWaypointsX(minIndex+1)-RefWaypointsX(minIndex);
constant=(delta_y)/(delta_x);
LineHeadingError=atan(constant);

HeadingError = LineHeadingError-convert_Theta; % [rad]
if abs(HeadingError) > 2.5
    if convert_Theta > 0 && LineHeadingError < 0
        HeadingError = pi-convert_Theta-LineHeadingError;
    end
    if convert_Theta < 0 && LineHeadingError >0
        HeadingError = LineHeadingError-convert_Theta-pi;
        
    end
    if convert_Theta > 0 && LineHeadingError < 0 && deriv_y <0
        HeadingError = -LineHeadingError-convert_Theta;
    end
end
e = abs((a*CurrX+CurrY+c)/(sqrt(a*a+1))); % CrossTrackError [m]
if isnan(e)
    e = RefWaypointsX(minIndex)-CurrX;
end
if abs(e)<0.0001
    e=0;
end
if abs(HeadingError)<0.0001
    HeadingError= 0;
end
% TotalSteering [rad] Needed steering angle for correct the orientation of
% the vehicle
Test = a*CurrX+CurrY+c; % Checks the position of the CurrPoint w.r.t line
Test2 = RefWaypointsX(minIndex)-CurrX;
Test3= RefWaypointsY(minIndex)-CurrY;
if isnan(Test)
    Test=Test2;
end
%% SPECIAL CASE 0<x<pi/2
if 0<LineHeadingError<pi/2
    if Test>0
        if deriv_y>0
            e=-abs(e);
        else
            e=abs(e);
        end
    else
        if deriv_y>0
            e=abs(e);
        else
            e=-abs(e);
        end
    end
end
%% SPECIAL CASE x==pi/2 or x==-pi/2

if LineHeadingError==pi/2 || LineHeadingError==-pi/2
    if Test2>0
        if deriv_y>0
            e=-abs(e);
        else
            e=abs(e);
        end
    else
        if deriv_y>0
            e=abs(e);
        else
            e=-abs(e);
        end
    end
end
%% SPECIAL CASE x==0

if LineHeadingError==0
    if Test3>0
        if deriv_x>0
            e=abs(e);
        else
            e=-abs(e);
        end
    else
        if deriv_x>0
            e=-abs(e);
        else
            e=abs(e);
        end
    end
end
%% SPECIAL CASE -pi/2<x<0
if -pi/2<LineHeadingError && LineHeadingError<0
    if Test>0
        if deriv_y>0
            e=abs(e);
        else
            e=-abs(e);
        end
    else
        if deriv_y>0
            e=-abs(e);
        else
            e=abs(e);
        end
    end
end



%if Test > 0
 %   e = -e;
%end

CrossTrackSteering = atan((k*e)/(WheelVelocity)); % [rad]

TotalSteering = HeadingError+CrossTrackSteering; % [rad]

== matlab function ControlSystem/CONTROL/MATLAB Function2 ==
  data: CurrX input; EstimatedVel output; CurrXPrev input; CurrY input; CurrYPrev input
function EstimatedVel = fcn(CurrX,CurrXPrev,CurrY,CurrYPrev)

EstimatedVel = (sqrt((CurrX-CurrXPrev)^2+(CurrY-CurrYPrev)^2))/0.01;

== matlab function ControlSystem/CONTROL/MATLAB Function ==
  data: LocalWaypointsX input; RefVelocity output; LocalWaypointsY input; start_speed input; desired_speed input; a_max input; closest_index input
function RefVelocity = fcn(LocalWaypointsX,LocalWaypointsY,start_speed,desired_speed,a_max,closest_index)

% function [profile] =
% fcn(RefWaypointsX,RefWaypointsY,start_speed,desired_speed) calculates the
% velocity profile
max_speed = 0.5;
if start_speed > max_speed
    RefVelocity = desired_speed;
    return 
end
Profile = zeros(1,length(LocalWaypointsX));
if desired_speed < start_speed
    accel_distance = -(desired_speed^2-start_speed^2)/(2*a_max);
else
    accel_distance = (desired_speed^2-start_speed^2)/(2*a_max);
end

ramp_end_index = 1;
distance = 0;

while ramp_end_index < length(LocalWaypointsX)-1 && accel_distance > distance
    distance = distance+sqrt((LocalWaypointsX(ramp_end_index+1)-LocalWaypointsX(ramp_end_index))^2+(LocalWaypointsY(ramp_end_index+1)-LocalWaypointsY(ramp_end_index))^2);
    ramp_end_index = ramp_end_index+1;
end


vi = start_speed;

for i=1:1:ramp_end_index
    dist = sqrt((LocalWaypointsX(i+1)-LocalWaypointsX(i))^2+(LocalWaypointsY(i+1)-LocalWaypointsY(i))^2);
    if desired_speed < start_speed
        vf = real(sqrt((vi*vi)-(2*a_max*dist)));
        if vf < desired_speed
            vf = desired_speed;
        end
    else
        vf = real(sqrt((vi*vi)+(2*a_max*dist)));
        if vf > desired_speed
            vf = desired_speed;
        end
    end
    Profile(i) = vi;    
    vi = vf;
end

for i=ramp_end_index+1:1:length(LocalWaypointsX)
    
    Profile(i) = desired_speed;
    
end

RefVelocity = Profile(closest_index);
end
%RefVelocity = 0.5;
